simulink model "TSR_Scenario_006_cs"  (Simulink 7.6)
settings: Solver=ode5  SolverMode=SingleTasking  StartTime=0.0  StopTime=inf  FixedStep=1/100  RelTol=1e-3
model workspace (MAT data in the model file):
  mbox_table : struct (value not decoded)
  model_closed = 0
  sim_status = 0
PreLoadFcn:
  | check_NUTS_defined;
  | 
  | assignin('base',['model_closed_' bdroot],false);
  | 
  | addpath('../includes_TSR/includes_TSR');
  | 
  | switch version('-release')
  | case {'2010a', '2010b', '2011a'}
  | addpath('../includes_TSR/ML2010b');
  | otherwise
  | addpath('../includes_TSR/ML2011b');
  | end
InitFcn:
  | PreScanExperimentInitFcn(bdroot)
StopFcn:
  | PreScanExperimentStopFcn(bdroot)
undefined symbols (not defined in the file): DiscIntNeverNeededParam, InitImageOutputDir, x_ini_VRML, y_ini_VRML, z_ini_VRML
libraries: simulink x36, PreScanSimulinkLibrary x25, simulink_extras x18, PreScanUsefulBlocks x7, simulink_need_slupdate x1
(part 1 of 10)
CloseFcn:
  | evalin('base',['clear model_closed_' bdroot]);
settings Model: Creator=PRESCAN  LastModifiedBy=buildbot
settings OptimizationCC: InitFltsAndDblsToZero=on
settings DebuggingCC: SaveWithParameterizedLinksMsg=none  SignalResolutionControl=TryResolveAllWithWarning  SolverPrmCheckMsg=none  MultiTaskDSMMsg=warning  MultiTaskCondExecSysMsg=none
settings SFSimCC: SimParseCustomCode=off
settings RTWCC: IncludeERTFirstTime=on
settings GRTTargetCC: TargetFcnLib=ansi_tfl_tmw.mat

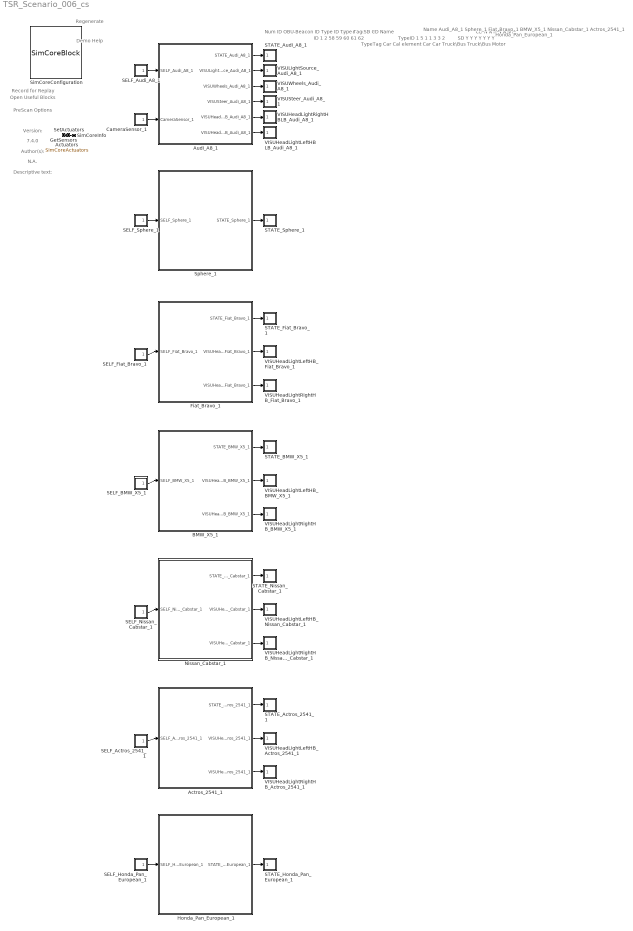
== system TSR_Scenario_006_cs ==
  note: Demo Help
  note: Regenerate
  note: Record for Replay
  note: Open Useful Blocks
  note: PreScan Options
  note: Version:
  note: 7.4.0
  note: Author(s):
  note: N.A.
  note: Descriptive text:
  note: ID
      |
      | 1
      | 2
      | 58
      | 59
      | 60
      | 61
      | 62
  note: OBU-Beacon ID
  note: TypeID
      |
      | 1
      | 5
      | 1
      | 1
      | 3
      | 3
      | 2
  note: TypeTag
      |
      | Car
      | Cal element
      | Car
      | Car
      | Truck\Bus
      | Truck\Bus
      | Motor
  note: SD
      |
      | Y
      | Y
      | Y
      | Y
      | Y
      | Y
      | Y
  note: CD
      |
      | N
      | N
      | N
      | N
      | N
      | N
      | N
  note: Name
      |
      | Audi_A8_1
      | Sphere_1
      | Fiat_Bravo_1
      | BMW_X5_1
      | Nissan_Cabstar_1
      | Actros_2541_1
      | Honda_Pan_European_1
  note: Num ID OBU-Beacon ID Type ID Type Tag SD CD Name
  Actros_2541_1 : Subsystem  Tag=WorldObjectSubSystem  InitFcn=UniqueId = '3230';
      mask Display: image(imread('Actros_2541.png'));color('white');text(0,0,' ID=61\n')
  Actuators : DataStoreMemory  Tag=Actuators  DataStoreName=SimCoreActuators  InitialValue=zeros(571,1)
      settings: DeleteFcn=PreScanBlockDeleteFcn;
  Audi_A8_1 : Subsystem  Tag=WorldObjectSubSystem  InitFcn=UniqueId = '253';
      mask Display: image(imread('Audi_A8.jpg'));color('white');text(0,0,' ID=1\n')
  BMW_X5_1 : Subsystem  Tag=WorldObjectSubSystem  InitFcn=UniqueId = '3222';
      mask Display: image(imread('BMW_X5.jpg'));color('white');text(0,0,' ID=59\n')
  CameraSensor_1 : Subsystem  Tag=CameraSensor  Priority=3
      settings: DeleteFcn=PreScanBlockDeleteFcn;
      mask Type: PreScan Source Block: Camera Sensor
      mask Description: The Camera Sensor provides a color or monochrome image.
      mask Help: eval('openHelp(457)')
      mask Display: image(imread('CameraSensor.png'))
  Fiat_Bravo_1 : Subsystem  Tag=WorldObjectSubSystem  InitFcn=UniqueId = '3219';
      mask Display: image(imread('Fiat_Bravo.jpg'));color('white');text(0,0,' ID=58\n')
  GetSensors : Subsystem  Tag=GetSensors  Priority=2  mask(PreScan Simulation Core Block){NrOfSensors=56, TimeStep=1/100}
      mask prompts: NrOfSensors "Number of sensor values"; TimeStep "Timestep [s]"
      mask help:
      | Please do not remove this block from the PreScan compilation sheet,
      | as it contains essential configuration parameters for a PreScan simulation.
      settings: DeleteFcn=PreScanBlockDeleteFcn;
  Honda_Pan_European_1 : Subsystem  Tag=WorldObjectSubSystem  InitFcn=UniqueId = '3233';
      mask Display: image(imread('Honda_Pan_European.jpg'));color('white');text(0,0,' ID=62\n')
  Nissan_Cabstar_1 : Subsystem  Tag=WorldObjectSubSystem  InitFcn=UniqueId = '3227';
      mask Display: image(imread('Nissan_Cabstar.jpg'));color('white');text(0,0,' ID=60\n')
  SELF_Actros_2541_1 : Subsystem  Tag=SELF  Priority=3  mask(PreScan Source Block: SELF){PortName=SELF_Actros_2541_1, PortIndex=40, PortWidth=8, TimeStep=1/100}
      mask prompts: PortName "Auto-Assigned: Port Name [-]"; PortIndex "Auto-Assigned: Port Index [-]"; PortWidth "Auto-Assigned: Port Dimensions"; TimeStep "Auto-Assigned: Upload Period [s]"
      mask help:
      | The SELF port shows (state) information of the actor itself. The outputs are position in the experiment's axis system and the GPS coordinates, and the object's absolute velocity and compass heading.
      |
      | For more information, please click Help.
      settings: DeleteFcn=PreScanBlockDeleteFcn;
      mask Help: eval('openHelp(462)')
      mask Display: image(imread('GPS.png'))
  SELF_Audi_A8_1 : Subsystem  Tag=SELF  Priority=3  mask(PreScan Source Block: SELF){PortName=SELF_Audi_A8_1, PortIndex=0, PortWidth=8, TimeStep=1/100}
      mask prompts: PortName "Auto-Assigned: Port Name [-]"; PortIndex "Auto-Assigned: Port Index [-]"; PortWidth "Auto-Assigned: Port Dimensions"; TimeStep "Auto-Assigned: Upload Period [s]"
      mask help:
      | The SELF port shows (state) information of the actor itself. The outputs are position in the experiment's axis system and the GPS coordinates, and the object's absolute velocity and compass heading.
      |
      | For more information, please click Help.
      settings: DeleteFcn=PreScanBlockDeleteFcn;
      mask Help: eval('openHelp(462)')
      mask Display: image(imread('GPS.png'))
  SELF_BMW_X5_1 : Subsystem  Tag=SELF  Priority=3  mask(PreScan Source Block: SELF){PortName=SELF_BMW_X5_1, PortIndex=24, PortWidth=8, TimeStep=1/100}
      mask prompts: PortName "Auto-Assigned: Port Name [-]"; PortIndex "Auto-Assigned: Port Index [-]"; PortWidth "Auto-Assigned: Port Dimensions"; TimeStep "Auto-Assigned: Upload Period [s]"
      mask help:
      | The SELF port shows (state) information of the actor itself. The outputs are position in the experiment's axis system and the GPS coordinates, and the object's absolute velocity and compass heading.
      |
      | For more information, please click Help.
      settings: DeleteFcn=PreScanBlockDeleteFcn;
      mask Help: eval('openHelp(462)')
      mask Display: image(imread('GPS.png'))
  SELF_Fiat_Bravo_1 : Subsystem  Tag=SELF  Priority=3  mask(PreScan Source Block: SELF){PortName=SELF_Fiat_Bravo_1, PortIndex=16, PortWidth=8, TimeStep=1/100}
      mask prompts: PortName "Auto-Assigned: Port Name [-]"; PortIndex "Auto-Assigned: Port Index [-]"; PortWidth "Auto-Assigned: Port Dimensions"; TimeStep "Auto-Assigned: Upload Period [s]"
      mask help:
      | The SELF port shows (state) information of the actor itself. The outputs are position in the experiment's axis system and the GPS coordinates, and the object's absolute velocity and compass heading.
      |
      | For more information, please click Help.
      settings: DeleteFcn=PreScanBlockDeleteFcn;
      mask Help: eval('openHelp(462)')
      mask Display: image(imread('GPS.png'))
  SELF_Honda_Pan_European_1 : Subsystem  Tag=SELF  Priority=3  mask(PreScan Source Block: SELF){PortName=SELF_Honda_Pan_European_1, PortIndex=48, PortWidth=8, TimeStep=1/100}
      mask prompts: PortName "Auto-Assigned: Port Name [-]"; PortIndex "Auto-Assigned: Port Index [-]"; PortWidth "Auto-Assigned: Port Dimensions"; TimeStep "Auto-Assigned: Upload Period [s]"
      mask help:
      | The SELF port shows (state) information of the actor itself. The outputs are position in the experiment's axis system and the GPS coordinates, and the object's absolute velocity and compass heading.
      |
      | For more information, please click Help.
      settings: DeleteFcn=PreScanBlockDeleteFcn;
      mask Help: eval('openHelp(462)')
      mask Display: image(imread('GPS.png'))
  SELF_Nissan_Cabstar_1 : Subsystem  Tag=SELF  Priority=3  mask(PreScan Source Block: SELF){PortName=SELF_Nissan_Cabstar_1, PortIndex=32, PortWidth=8, TimeStep=1/100}
      mask prompts: PortName "Auto-Assigned: Port Name [-]"; PortIndex "Auto-Assigned: Port Index [-]"; PortWidth "Auto-Assigned: Port Dimensions"; TimeStep "Auto-Assigned: Upload Period [s]"
      mask help:
      | The SELF port shows (state) information of the actor itself. The outputs are position in the experiment's axis system and the GPS coordinates, and the object's absolute velocity and compass heading.
      |
      | For more information, please click Help.
      settings: DeleteFcn=PreScanBlockDeleteFcn;
      mask Help: eval('openHelp(462)')
      mask Display: image(imread('GPS.png'))
  SELF_Sphere_1 : Subsystem  Tag=SELF  Priority=3  mask(PreScan Source Block: SELF){PortName=SELF_Sphere_1, PortIndex=8, PortWidth=8, TimeStep=1/100}
      mask prompts: PortName "Auto-Assigned: Port Name [-]"; PortIndex "Auto-Assigned: Port Index [-]"; PortWidth "Auto-Assigned: Port Dimensions"; TimeStep "Auto-Assigned: Upload Period [s]"
      mask help:
      | The SELF port shows (state) information of the actor itself. The outputs are position in the experiment's axis system and the GPS coordinates, and the object's absolute velocity and compass heading.
      |
      | For more information, please click Help.
      settings: DeleteFcn=PreScanBlockDeleteFcn;
      mask Help: eval('openHelp(462)')
      mask Display: image(imread('GPS.png'))
  STATE_Actros_2541_1 : Subsystem  Tag=State  Priority=0  mask(PreScan Sink Block: State){x0=-317.51490220295977, y0=442.15687795747425, z0=0.6, Roll0=0, Pitch0=0, Yaw0=329.99999999999994, TimeStep=1/100}
      mask prompts: x0 "Ini x-position VEHICLE wrt GLOBAL axis system [m]"; y0 "Ini y-position VEHICLE wrt GLOBAL axis system [m]"; z0 "Ini z-position VEHICLE wrt GLOBAL axis system [m]"; Roll0 "Ini roll-angle BODY wrt VEHICLE axis system [deg]"; Pitch0 "Ini pitch-angle BODY wrt VEHICLE axis system [deg]"; Yaw0 "Ini yaw-angle VEHICLE wrt GLOBAL axis system [deg]"; TimeStep "Time Step [s]"
      mask help:
      | The Actor State contains a vector signal of size (9x1), containing the following signals:
      |
      | -  Position                  (x,y,z)                                     [m]
      | -  Velocity                  (vx,vy,vz)                               [m/s]
      | -  Angles                    (Roll, Pitch, Yaw)                   [rad]
      |
      | The Actor state is defined in the global axis system.
      | The state is superponed on the Initial position defined in the GUI.
      |
      | For more information, please click Help.
      settings: DeleteFcn=PreScanBlockDeleteFcn;
      mask Help: eval('openHelp(222)')
      mask Display: image(imread('State.png'))
  STATE_Audi_A8_1 : Subsystem  Tag=State  Priority=0  mask(PreScan Sink Block: State){x0=-413.08909402600443, y0=672.31264940005644, z0=0.55, Roll0=0, Pitch0=0, Yaw0=19.15644857361562, TimeStep=1/100}
      mask prompts: x0 "Ini x-position VEHICLE wrt GLOBAL axis system [m]"; y0 "Ini y-position VEHICLE wrt GLOBAL axis system [m]"; z0 "Ini z-position VEHICLE wrt GLOBAL axis system [m]"; Roll0 "Ini roll-angle BODY wrt VEHICLE axis system [deg]"; Pitch0 "Ini pitch-angle BODY wrt VEHICLE axis system [deg]"; Yaw0 "Ini yaw-angle VEHICLE wrt GLOBAL axis system [deg]"; TimeStep "Time Step [s]"
      mask help:
      | The Actor State contains a vector signal of size (9x1), containing the following signals:
      |
      | -  Position                  (x,y,z)                                     [m]
      | -  Velocity                  (vx,vy,vz)                               [m/s]
      | -  Angles                    (Roll, Pitch, Yaw)                   [rad]
      |
      | The Actor state is defined in the global axis system.
      | The state is superponed on the Initial position defined in the GUI.
      |
      | For more information, please click Help.
      settings: DeleteFcn=PreScanBlockDeleteFcn;
      mask Help: eval('openHelp(222)')
      mask Display: image(imread('State.png'))
  STATE_BMW_X5_1 : Subsystem  Tag=State  Priority=0  mask(PreScan Sink Block: State){x0=-278.56622618717029, y0=100.14255486855011, z0=0.69, Roll0=0, Pitch0=0, Yaw0=248.31002382560104, TimeStep=1/100}
      mask prompts: x0 "Ini x-position VEHICLE wrt GLOBAL axis system [m]"; y0 "Ini y-position VEHICLE wrt GLOBAL axis system [m]"; z0 "Ini z-position VEHICLE wrt GLOBAL axis system [m]"; Roll0 "Ini roll-angle BODY wrt VEHICLE axis system [deg]"; Pitch0 "Ini pitch-angle BODY wrt VEHICLE axis system [deg]"; Yaw0 "Ini yaw-angle VEHICLE wrt GLOBAL axis system [deg]"; TimeStep "Time Step [s]"
      mask help:
      | The Actor State contains a vector signal of size (9x1), containing the following signals:
      |
      | -  Position                  (x,y,z)                                     [m]
      | -  Velocity                  (vx,vy,vz)                               [m/s]
      | -  Angles                    (Roll, Pitch, Yaw)                   [rad]
      |
      | The Actor state is defined in the global axis system.
      | The state is superponed on the Initial position defined in the GUI.
      |
      | For more information, please click Help.
      settings: DeleteFcn=PreScanBlockDeleteFcn;
      mask Help: eval('openHelp(222)')
      mask Display: image(imread('State.png'))
  STATE_Fiat_Bravo_1 : Subsystem  Tag=State  Priority=0  mask(PreScan Sink Block: State){x0=-278.56622618717029, y0=100.14255486855011, z0=0.55, Roll0=0, Pitch0=0, Yaw0=248.31002382560104, TimeStep=1/100}
      mask prompts: x0 "Ini x-position VEHICLE wrt GLOBAL axis system [m]"; y0 "Ini y-position VEHICLE wrt GLOBAL axis system [m]"; z0 "Ini z-position VEHICLE wrt GLOBAL axis system [m]"; Roll0 "Ini roll-angle BODY wrt VEHICLE axis system [deg]"; Pitch0 "Ini pitch-angle BODY wrt VEHICLE axis system [deg]"; Yaw0 "Ini yaw-angle VEHICLE wrt GLOBAL axis system [deg]"; TimeStep "Time Step [s]"
      mask help:
      | The Actor State contains a vector signal of size (9x1), containing the following signals:
      |
      | -  Position                  (x,y,z)                                     [m]
      | -  Velocity                  (vx,vy,vz)                               [m/s]
      | -  Angles                    (Roll, Pitch, Yaw)                   [rad]
      |
      | The Actor state is defined in the global axis system.
      | The state is superponed on the Initial position defined in the GUI.
      |
      | For more information, please click Help.
      settings: DeleteFcn=PreScanBlockDeleteFcn;
      mask Help: eval('openHelp(222)')
      mask Display: image(imread('State.png'))
  STATE_Honda_Pan_European_1 : Subsystem  Tag=State  Priority=0  mask(PreScan Sink Block: State){x0=-295.55667114257812, y0=275.828369140625, z0=0.594, Roll0=0, Pitch0=0, Yaw0=330, TimeStep=1/100}
      mask prompts: x0 "Ini x-position VEHICLE wrt GLOBAL axis system [m]"; y0 "Ini y-position VEHICLE wrt GLOBAL axis system [m]"; z0 "Ini z-position VEHICLE wrt GLOBAL axis system [m]"; Roll0 "Ini roll-angle BODY wrt VEHICLE axis system [deg]"; Pitch0 "Ini pitch-angle BODY wrt VEHICLE axis system [deg]"; Yaw0 "Ini yaw-angle VEHICLE wrt GLOBAL axis system [deg]"; TimeStep "Time Step [s]"
      mask help:
      | The Actor State contains a vector signal of size (9x1), containing the following signals:
      |
      | -  Position                  (x,y,z)                                     [m]
      | -  Velocity                  (vx,vy,vz)                               [m/s]
      | -  Angles                    (Roll, Pitch, Yaw)                   [rad]
      |
      | The Actor state is defined in the global axis system.
      | The state is superponed on the Initial position defined in the GUI.
      |
      | For more information, please click Help.
      settings: DeleteFcn=PreScanBlockDeleteFcn;
      mask Help: eval('openHelp(222)')
      mask Display: image(imread('State.png'))
  STATE_Nissan_Cabstar_1 : Subsystem  Tag=State  Priority=0  mask(PreScan Sink Block: State){x0=-125.23931337038341, y0=335.18796687071978, z0=0.88, Roll0=0, Pitch0=0, Yaw0=150, TimeStep=1/100}
      mask prompts: x0 "Ini x-position VEHICLE wrt GLOBAL axis system [m]"; y0 "Ini y-position VEHICLE wrt GLOBAL axis system [m]"; z0 "Ini z-position VEHICLE wrt GLOBAL axis system [m]"; Roll0 "Ini roll-angle BODY wrt VEHICLE axis system [deg]"; Pitch0 "Ini pitch-angle BODY wrt VEHICLE axis system [deg]"; Yaw0 "Ini yaw-angle VEHICLE wrt GLOBAL axis system [deg]"; TimeStep "Time Step [s]"
      mask help:
      | The Actor State contains a vector signal of size (9x1), containing the following signals:
      |
      | -  Position                  (x,y,z)                                     [m]
      | -  Velocity                  (vx,vy,vz)                               [m/s]
      | -  Angles                    (Roll, Pitch, Yaw)                   [rad]
      |
      | The Actor state is defined in the global axis system.
      | The state is superponed on the Initial position defined in the GUI.
      |
      | For more information, please click Help.
      settings: DeleteFcn=PreScanBlockDeleteFcn;
      mask Help: eval('openHelp(222)')
      mask Display: image(imread('State.png'))
  STATE_Sphere_1 : Subsystem  Tag=State  Priority=0  mask(PreScan Sink Block: State){x0=-413.089094026004, y0=672.312649400056, z0=0.55, Roll0=0, Pitch0=0, Yaw0=19.1564485736156, TimeStep=1/100}
      mask prompts: x0 "Ini x-position VEHICLE wrt GLOBAL axis system [m]"; y0 "Ini y-position VEHICLE wrt GLOBAL axis system [m]"; z0 "Ini z-position VEHICLE wrt GLOBAL axis system [m]"; Roll0 "Ini roll-angle BODY wrt VEHICLE axis system [deg]"; Pitch0 "Ini pitch-angle BODY wrt VEHICLE axis system [deg]"; Yaw0 "Ini yaw-angle VEHICLE wrt GLOBAL axis system [deg]"; TimeStep "Time Step [s]"
      mask help:
      | The Actor State contains a vector signal of size (9x1), containing the following signals:
      |
      | -  Position                  (x,y,z)                                     [m]
      | -  Velocity                  (vx,vy,vz)                               [m/s]
      | -  Angles                    (Roll, Pitch, Yaw)                   [rad]
      |
      | The Actor state is defined in the global axis system.
      | The state is superponed on the Initial position defined in the GUI.
      |
      | For more information, please click Help.
      settings: DeleteFcn=PreScanBlockDeleteFcn;
      mask Help: eval('openHelp(222)')
      mask Display: image(imread('State.png'))
  SetActuators : Subsystem  Tag=SetActuators  Priority=1  mask(PreScan Simulation Core Block){TimeStep=1/100, NrOfActuators=571}
      mask prompts: TimeStep "Timestep [s]"; NrOfActuators "Number of actuator values"
      mask help:
      | Please do not remove this block from the PreScan compilation sheet,
      | as it contains essential configuration parameters for a PreScan simulation.
      settings: DeleteFcn=PreScanBlockDeleteFcn;
  SimCoreConfiguration : M-S-Function  Tag=SimCoreConfiguration  Description=313268978F12D5AD1759FB37E42A829EE63F37BD296FA7458A7FCDBDC14E6B1E  FunctionName=SimCoreBlock  Parameters=ExperimentXML PortsXML SimulationCore HostName CheckStart EnableLog RfR EnableGPUAccel ShowComputationTime  mask(PreScan Simulation Core Configurator){SimulationCore=NUTS, HostName=0, CheckStart=0, prescanversion='7.4.0', EnableLog=off, RfR=0, EnableGPUAccel=off, ShowComputationTime=off}
      mask prompts: SimulationCore "Simulation Core"; HostName "Simulation Host"; CheckStart "Show START Dialog"; prescanversion "PreScan Version"; EnableLog "Create TA Log"; RfR "Record for Replay"; EnableGPUAccel "Enable GPU Acceleration"; ShowComputationTime "Show ComputationTime Scope"
      mask help:
      | Please do not remove this block from the PreScan compilation sheet,
      | as it contains essential configuration parameter for a PreScan simulation.
      mask init:
      | model = bdroot;
      | ExperimentXML = [model(1:end-3) '.pex'];
      | PortsXML = [model '_ports.pcd'];
      settings: DeleteFcn=PreScanBlockDeleteFcn;  ModelCloseFcn=assignin('base',['model_closed_' bdroot],true);
      mask Help: eval('openHelp(812)')
      mask Display: image(imread('prescanlogo.ico'))
  SimCoreInfo : Subsystem  Tag=SimCoreInfo
  Sphere_1 : Subsystem  Tag=WorldObjectSubSystem  InitFcn=UniqueId = '277';
      mask Display: image(imread('Sphere.jpg'));color('white');text(0,0,' ID=2\n')
  VISUHeadLightLeftHBLB_Audi_A8_1 : Subsystem  Tag=VisuLights  Priority=0
      settings: DeleteFcn=PreScanBlockDeleteFcn;
      mask Type: PreScan Sink Block: VisuLights
      mask Description:
      | The VisuLights block provides a way to animate the active lights of a vehicle with possibilities to adapt the:
      | - Intensity [-]
      | - Position (x,y,z) [m]
      | - Orientation (Roll, Pitch, Yaw) [deg]
      | - Color (RGB) [-]
      | - TextureResourceID [-]
      | 
      | For more information, please click Help.
      mask Help: eval('openHelp(231)')
      mask Display: image(imread('HeadLight.png'))
  VISUHeadLightLeftHB_Actros_2541_1 : Subsystem  Tag=VisuLights  Priority=0
      settings: DeleteFcn=PreScanBlockDeleteFcn;
      mask Type: PreScan Sink Block: VisuLights
      mask Description:
      | The VisuLights block provides a way to animate the active lights of a vehicle with possibilities to adapt the:
      | - Intensity [-]
      | - Position (x,y,z) [m]
      | - Orientation (Roll, Pitch, Yaw) [deg]
      | - Color (RGB) [-]
      | - TextureResourceID [-]
      | 
      | For more information, please click Help.
      mask Help: eval('openHelp(231)')
      mask Display: image(imread('HeadLight.png'))
  VISUHeadLightLeftHB_BMW_X5_1 : Subsystem  Tag=VisuLights  Priority=0
      settings: DeleteFcn=PreScanBlockDeleteFcn;
      mask Type: PreScan Sink Block: VisuLights
      mask Description:
      | The VisuLights block provides a way to animate the active lights of a vehicle with possibilities to adapt the:
      | - Intensity [-]
      | - Position (x,y,z) [m]
      | - Orientation (Roll, Pitch, Yaw) [deg]
      | - Color (RGB) [-]
      | - TextureResourceID [-]
      | 
      | For more information, please click Help.
      mask Help: eval('openHelp(231)')
      mask Display: image(imread('HeadLight.png'))
  VISUHeadLightLeftHB_Fiat_Bravo_1 : Subsystem  Tag=VisuLights  Priority=0
      settings: DeleteFcn=PreScanBlockDeleteFcn;
      mask Type: PreScan Sink Block: VisuLights
      mask Description:
      | The VisuLights block provides a way to animate the active lights of a vehicle with possibilities to adapt the:
      | - Intensity [-]
      | - Position (x,y,z) [m]
      | - Orientation (Roll, Pitch, Yaw) [deg]
      | - Color (RGB) [-]
      | - TextureResourceID [-]
      | 
      | For more information, please click Help.
      mask Help: eval('openHelp(231)')
      mask Display: image(imread('HeadLight.png'))
  VISUHeadLightLeftHB_Nissan_Cabstar_1 : Subsystem  Tag=VisuLights  Priority=0
      settings: DeleteFcn=PreScanBlockDeleteFcn;
      mask Type: PreScan Sink Block: VisuLights
      mask Description:
      | The VisuLights block provides a way to animate the active lights of a vehicle with possibilities to adapt the:
      | - Intensity [-]
      | - Position (x,y,z) [m]
      | - Orientation (Roll, Pitch, Yaw) [deg]
      | - Color (RGB) [-]
      | - TextureResourceID [-]
      | 
      | For more information, please click Help.
      mask Help: eval('openHelp(231)')
      mask Display: image(imread('HeadLight.png'))
  VISUHeadLightRightHBLB_Audi_A8_1 : Subsystem  Tag=VisuLights  Priority=0
      settings: DeleteFcn=PreScanBlockDeleteFcn;
      mask Type: PreScan Sink Block: VisuLights
      mask Description:
      | The VisuLights block provides a way to animate the active lights of a vehicle with possibilities to adapt the:
      | - Intensity [-]
      | - Position (x,y,z) [m]
      | - Orientation (Roll, Pitch, Yaw) [deg]
      | - Color (RGB) [-]
      | - TextureResourceID [-]
      | 
      | For more information, please click Help.
      mask Help: eval('openHelp(231)')
      mask Display: image(imread('HeadLight.png'))
  VISUHeadLightRightHB_Actros_2541_1 : Subsystem  Tag=VisuLights  Priority=0
      settings: DeleteFcn=PreScanBlockDeleteFcn;
      mask Type: PreScan Sink Block: VisuLights
      mask Description:
      | The VisuLights block provides a way to animate the active lights of a vehicle with possibilities to adapt the:
      | - Intensity [-]
      | - Position (x,y,z) [m]
      | - Orientation (Roll, Pitch, Yaw) [deg]
      | - Color (RGB) [-]
      | - TextureResourceID [-]
      | 
      | For more information, please click Help.
      mask Help: eval('openHelp(231)')
      mask Display: image(imread('HeadLight.png'))
  VISUHeadLightRightHB_BMW_X5_1 : Subsystem  Tag=VisuLights  Priority=0
      settings: DeleteFcn=PreScanBlockDeleteFcn;
      mask Type: PreScan Sink Block: VisuLights
      mask Description:
      | The VisuLights block provides a way to animate the active lights of a vehicle with possibilities to adapt the:
      | - Intensity [-]
      | - Position (x,y,z) [m]
      | - Orientation (Roll, Pitch, Yaw) [deg]
      | - Color (RGB) [-]
      | - TextureResourceID [-]
      | 
      | For more information, please click Help.
      mask Help: eval('openHelp(231)')
      mask Display: image(imread('HeadLight.png'))
  VISUHeadLightRightHB_Fiat_Bravo_1 : Subsystem  Tag=VisuLights  Priority=0
      settings: DeleteFcn=PreScanBlockDeleteFcn;
      mask Type: PreScan Sink Block: VisuLights
      mask Description:
      | The VisuLights block provides a way to animate the active lights of a vehicle with possibilities to adapt the:
      | - Intensity [-]
      | - Position (x,y,z) [m]
      | - Orientation (Roll, Pitch, Yaw) [deg]
      | - Color (RGB) [-]
      | - TextureResourceID [-]
      | 
      | For more information, please click Help.
      mask Help: eval('openHelp(231)')
      mask Display: image(imread('HeadLight.png'))
  VISUHeadLightRightHB_Nissan_Cabstar_1 : Subsystem  Tag=VisuLights  Priority=0
      settings: DeleteFcn=PreScanBlockDeleteFcn;
      mask Type: PreScan Sink Block: VisuLights
      mask Description:
      | The VisuLights block provides a way to animate the active lights of a vehicle with possibilities to adapt the:
      | - Intensity [-]
      | - Position (x,y,z) [m]
      | - Orientation (Roll, Pitch, Yaw) [deg]
      | - Color (RGB) [-]
      | - TextureResourceID [-]
      | 
      | For more information, please click Help.
      mask Help: eval('openHelp(231)')
      mask Display: image(imread('HeadLight.png'))
  VISULightSource_Audi_A8_1 : Subsystem  Tag=VisuLightSource  Priority=0
      settings: DeleteFcn=PreScanBlockDeleteFcn;
      mask Type: PreScan Sink Block: VisuLightSource
      mask Description:
      | The VisuLightSource block provides a way to animate Light Sources of the indicator, braking, fog and main lights of a vehicle.
      | 
      | For more information, please click Help.
      mask Help: eval('openHelp(223)')
      mask Display: image(imread('RearLight.png'))
  VISUSteer_Audi_A8_1 : Subsystem  Tag=VisuSteer  Priority=0
      settings: DeleteFcn=PreScanBlockDeleteFcn;
      mask Type: PreScan Sink Block: VisuSteer
      mask Description:
      | The VisuSteer block provides a way to adapt the orientation of the steering column and steering wheel of a vehicle.
      | 
      | For more information, please click Help.
      mask Help: eval('openHelp(223)')
      mask Display: image(imread('steeringwheel.png'))
  VISUWheels_Audi_A8_1 : Subsystem  Tag=VisuWheels  Priority=0
      settings: DeleteFcn=PreScanBlockDeleteFcn;
      mask Type: PreScan Sink Block: VisuWheels
      mask Description:
      | The VisuWheels block provides a way to animate the wheels of a vehicle, with steering, rotation (because of velocity) and z-displacement.
      | 
      | For more information, please click Help.
      mask Help: eval('openHelp(223)')
      mask Display: image(imread('wheel.png'))
  wires:
  Audi_A8_1/1(STATE_Audi_A8_1) -> STATE_Audi_A8_1/1(State)
  SELF_Audi_A8_1/1(U) -> Audi_A8_1/1(SELF_Audi_A8_1)
  CameraSensor_1/1(U1) -> Audi_A8_1/2(CameraSensor_1)
  Audi_A8_1/2(VISULightSource_Audi_A8_1) -> VISULightSource_Audi_A8_1/1(Lights)
  Audi_A8_1/3(VISUWheels_Audi_A8_1) -> VISUWheels_Audi_A8_1/1(Wheels)
  Audi_A8_1/4(VISUSteer_Audi_A8_1) -> VISUSteer_Audi_A8_1/1(Steer)
  Audi_A8_1/5(VISUHeadLightRightHBLB_Audi_A8_1) -> VISUHeadLightRightHBLB_Audi_A8_1/1(Lights)
  Audi_A8_1/6(VISUHeadLightLeftHBLB_Audi_A8_1) -> VISUHeadLightLeftHBLB_Audi_A8_1/1(Lights)
  Sphere_1/1(STATE_Sphere_1) -> STATE_Sphere_1/1(State)
  SELF_Sphere_1/1(U) -> Sphere_1/1(SELF_Sphere_1)
  Fiat_Bravo_1/1(STATE_Fiat_Bravo_1) -> STATE_Fiat_Bravo_1/1(State)
  SELF_Fiat_Bravo_1/1(U) -> Fiat_Bravo_1/1(SELF_Fiat_Bravo_1)
  Fiat_Bravo_1/2(VISUHeadLightLeftHB_Fiat_Bravo_1) -> VISUHeadLightLeftHB_Fiat_Bravo_1/1(Lights)
  Fiat_Bravo_1/3(VISUHeadLightRightHB_Fiat_Bravo_1) -> VISUHeadLightRightHB_Fiat_Bravo_1/1(Lights)
  BMW_X5_1/1(STATE_BMW_X5_1) -> STATE_BMW_X5_1/1(State)
  SELF_BMW_X5_1/1(U) -> BMW_X5_1/1(SELF_BMW_X5_1)
  BMW_X5_1/2(VISUHeadLightLeftHB_BMW_X5_1) -> VISUHeadLightLeftHB_BMW_X5_1/1(Lights)
  BMW_X5_1/3(VISUHeadLightRightHB_BMW_X5_1) -> VISUHeadLightRightHB_BMW_X5_1/1(Lights)
  Nissan_Cabstar_1/1(STATE_Nissan_Cabstar_1) -> STATE_Nissan_Cabstar_1/1(State)
  SELF_Nissan_Cabstar_1/1(U) -> Nissan_Cabstar_1/1(SELF_Nissan_Cabstar_1)
  Nissan_Cabstar_1/2(VISUHeadLightLeftHB_Nissan_Cabstar_1) -> VISUHeadLightLeftHB_Nissan_Cabstar_1/1(Lights)
  Nissan_Cabstar_1/3(VISUHeadLightRightHB_Nissan_Cabstar_1) -> VISUHeadLightRightHB_Nissan_Cabstar_1/1(Lights)
  Actros_2541_1/1(STATE_Actros_2541_1) -> STATE_Actros_2541_1/1(State)
  SELF_Actros_2541_1/1(U) -> Actros_2541_1/1(SELF_Actros_2541_1)
  Actros_2541_1/2(VISUHeadLightLeftHB_Actros_2541_1) -> VISUHeadLightLeftHB_Actros_2541_1/1(Lights)
  Actros_2541_1/3(VISUHeadLightRightHB_Actros_2541_1) -> VISUHeadLightRightHB_Actros_2541_1/1(Lights)
  Honda_Pan_European_1/1(STATE_Honda_Pan_European_1) -> STATE_Honda_Pan_European_1/1(State)
  SELF_Honda_Pan_European_1/1(U) -> Honda_Pan_European_1/1(SELF_Honda_Pan_European_1)
  SetActuators/1(dummy) -> GetSensors/1(dummy)

== system TSR_Scenario_006_cs/Actros_2541_1 ==
  note: Resources
      |
      | 1: LightMap\HeadLight LB and HB.png: HeadLight LB and HB
      | 2: LightMap\HeadLight HB.png: HeadLight HB
  note: Resources
  SELF_Actros_2541_1 : Inport  Tag=SELFInport
  HeadLightLeftHB_Col : Constant  Tag=VisuLightConst  Value=[255 249 224]
  HeadLightLeftHB_ID : Constant  Tag=VisuLightConst  Value=[0]
  HeadLightLeftHB_Ori : Constant  Tag=VisuLightConst  Value=[0 2 358]
  HeadLightLeftHB_Pos : Constant  Tag=VisuLightConst  Value=[5.93481 1.00553 0.797323]
  HeadLightLeftHB_mscd : Constant  Tag=VisuLightConst  Value=[98.20]
  HeadLightRightHB_Col : Constant  Tag=VisuLightConst  Value=[255 249 224]
  HeadLightRightHB_ID : Constant  Tag=VisuLightConst  Value=[0]
  HeadLightRightHB_Ori : Constant  Tag=VisuLightConst  Value=[0 0 358]
  HeadLightRightHB_Pos : Constant  Tag=VisuLightConst  Value=[5.93481 -1.0055 0.797323]
  HeadLightRightHB_mscd : Constant  Tag=VisuLightConst  Value=[98.20]
  SELF_Demux : Subsystem  Tag=DemuxSELF
      settings: DeleteFcn=PreScanBlockDeleteFcn;
      mask Type: PreScan Demux Block:
      mask Display:
      | port_label('output',1,'x [m]')
      | port_label('output',2,'y [m]')
      | port_label('output',3,'z [m]','texmode','on')
      | port_label('output',4,'Rotx [deg]','texmode','on')
      | port_label('output',5,'Roty [deg]','texmode','on')
      | port_label('output',6,'Rotz [deg]','texmode','on')
      | port_label('output',7,'GPS lat [deg]','texmode','on')
      | port_label('output',8,'GPS long [deg]','texmode','on')
      | port_label('output',9,'GPS alt [m]','texmode','on')
      | port_label('output',10,'Velocity [m/s]')
      | port_label('output',11,'Heading [deg]')
      | port_label('output',12,'Yaw rate [deg/s]')
  Terminator_{1..12} (12 alike) : Terminator
  Trajectories : Subsystem  Tag=Trajectories
      settings: DeleteFcn=PreScanBlockDeleteFcn;
      mask Type: PreScan Source Block: Trajectories
      mask Description:
      | The Trajectory block contains the trajectories defined in the PreScan Experiment Editor. The output of the trajectory block is the (vehicle) State.
      | 
      | For more information, please click Help.
      mask Help: eval('openHelp(312)')
      mask Display: image(imread('Trajectory.png'));
  VISUHeadLightLeftHB_Mux : Subsystem  Tag=MuxLights
      settings: DeleteFcn=PreScanBlockDeleteFcn;
      mask Type: PreScan Mux Block:
  VISUHeadLightRightHB_Mux : Subsystem  Tag=MuxLights
      settings: DeleteFcn=PreScanBlockDeleteFcn;
      mask Type: PreScan Mux Block:
  STATE_Actros_2541_1 : Outport  Tag=StateOutport
  VISUHeadLightLeftHB_Actros_2541_1 : Outport  Tag=VisuHeadLightLeftHBOutport  Port=2  SampleTime=1/100
  VISUHeadLightRightHB_Actros_2541_1 : Outport  Tag=VisuHeadLightRightHBOutport  Port=3  SampleTime=1/100
  wires:
  SELF_Actros_2541_1/1 -> SELF_Demux/1(SELF)
  VISUHeadLightLeftHB_Mux/1(Lights) -> VISUHeadLightLeftHB_Actros_2541_1/1
  HeadLightLeftHB_mscd/1 -> VISUHeadLightLeftHB_Mux/1(MSCD [Cd])
  HeadLightLeftHB_Pos/1 -> VISUHeadLightLeftHB_Mux/2(Position (xyz) [m])
  HeadLightLeftHB_Ori/1 -> VISUHeadLightLeftHB_Mux/3(Orientation (RPY) [deg])
  HeadLightLeftHB_Col/1 -> VISUHeadLightLeftHB_Mux/4(Color [-])
  HeadLightLeftHB_ID/1 -> VISUHeadLightLeftHB_Mux/5(TextureResourceID [-])
  VISUHeadLightRightHB_Mux/1(Lights) -> VISUHeadLightRightHB_Actros_2541_1/1
  HeadLightRightHB_mscd/1 -> VISUHeadLightRightHB_Mux/1(MSCD [Cd])
  HeadLightRightHB_Pos/1 -> VISUHeadLightRightHB_Mux/2(Position (xyz) [m])
  HeadLightRightHB_Ori/1 -> VISUHeadLightRightHB_Mux/3(Orientation (RPY) [deg])
  HeadLightRightHB_Col/1 -> VISUHeadLightRightHB_Mux/4(Color [-])
  HeadLightRightHB_ID/1 -> VISUHeadLightRightHB_Mux/5(TextureResourceID [-])
  Trajectories/1(State) -> STATE_Actros_2541_1/1
  SELF_Demux/1(x [m]) -> Terminator_1/1
  SELF_Demux/2(y [m]) -> Terminator_2/1
  SELF_Demux/3(z [m]) -> Terminator_3/1
  SELF_Demux/4(rotx [deg]) -> Terminator_4/1
  SELF_Demux/5(roty [deg]) -> Terminator_5/1
  SELF_Demux/6(rotz [deg]) -> Terminator_6/1
  SELF_Demux/7(GPS lat [deg]) -> Terminator_7/1
  SELF_Demux/8(GPS long [deg]) -> Terminator_8/1
  SELF_Demux/9(GPS alt [m]) -> Terminator_9/1
  SELF_Demux/10(velocity [m/s]) -> Terminator_10/1
  SELF_Demux/11(heading [deg]) -> Terminator_11/1
  SELF_Demux/12(yaw rate [deg/s]) -> Terminator_12/1

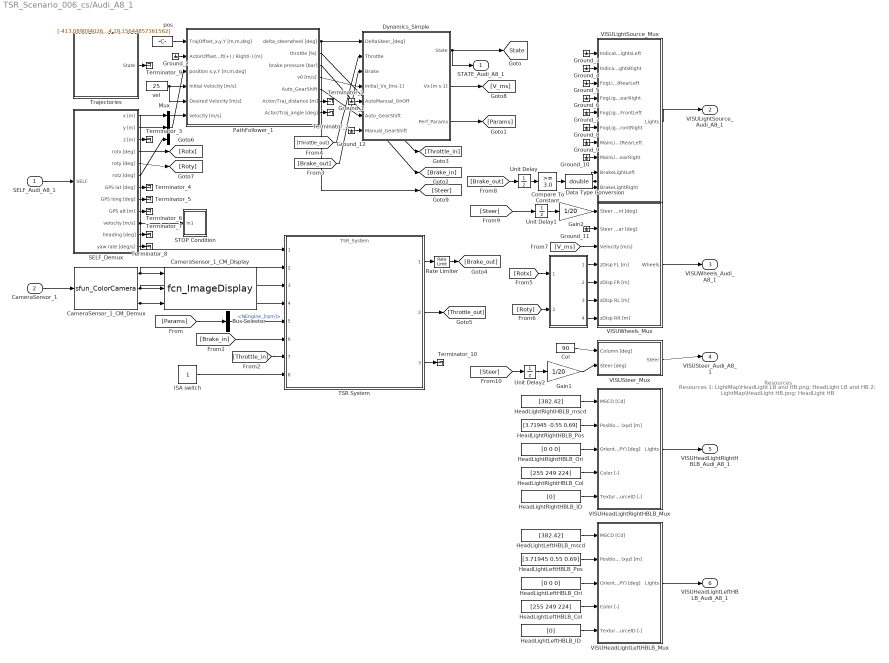
== system TSR_Scenario_006_cs/Audi_A8_1 ==
  note: Resources
      |
      | 1: LightMap\HeadLight LB and HB.png: HeadLight LB and HB
      | 2: LightMap\HeadLight HB.png: HeadLight HB
  note: Resources
  SELF_Audi_A8_1 : Inport  Tag=SELFInport
  CameraSensor_1 : Inport  Tag=CameraSensorInport  Port=2  SampleTime=1/50
  " " : Subsystem  mask{da=1.17, db=1.77, h=0.21, w=1.612}
      mask prompts: da "Distance to the front wheel from cars center of gravity [m]"; db "Distance to the back wheel from cars center of gravity [m]"; h "Center of gravity height [m]"; w "Width of the car [m]"
      mask init:
      | a  = sqrt( da*da + h*h );
      | b  = sqrt( db*db + h*h );
      | TW = sqrt( 0.25*w*w + h*h );
  Bus Selector : BusSelector  OutputSignals=NEngine_[rpm]
  CameraSensor_1_CM_Demux : S-Function  Tag=CameraSensor_Color_Demux  FunctionName=sfun_ColorCamera  Parameters=[VerticalResolution HorizontalResolution] FrameRate SensorName CameraType SharedMemTag SharedMemRightTag DataType  EnableBusSupport=off  mask{HorizontalResolution=800, VerticalResolution=600, FrameRate=50, SensorName=CameraSensor_1, CameraType=Mono, SharedMemTag=CameraSensor_1_monoBeam_viewer_RGB, SharedMemRightTag=CameraSensor_1_StereoRight_viewer_RGB, DataType=uint8}
      mask prompts: HorizontalResolution "User Specified: Horizontal Resolution [pixels]"; VerticalResolution "User Specified: Vertical Resolution [pixels]"; FrameRate "User Specified: Frame Rate [Hz]"; SensorName "User Specified: Camera Sensor Name"; CameraType "Camera Type"; SharedMemTag "Tag for shared memory for main img"; SharedMemRightTag "Tag for shared memory for right img"; DataType "Image Data Type"
      mask init:
      | if CameraType==1
      |     CameraTypeName='MONO';
      |     PortNumber=0;
      | else
      |     CameraTypeName='STEREO';
      |     PortNumber=3;
      | end
      settings: DeleteFcn=PreScanBlockDeleteFcn;
      mask StyleString: edit,edit,edit,edit,popup(Mono|Stereo),edit,edit,popup(uint8|single)
      mask Display:
      | fprintf('%s CAMERA:\n Color\n %s \n V: %d x %d \n %d fps',CameraTypeName,SensorName,VerticalResolution,HorizontalResolution,FrameRate)
      | port_label('output',1,'R')
      | port_label('output',2,'G')
      | port_label('output',3,'B')
      | port_label('output',PortNumber+1,'R')
      | port_label('output',PortNumber+2,'G')
      | port_label('output',PortNumber+3,'B')
  CameraSensor_1_CM_Display : M-S-Function  Tag=CameraSensor_Color_Display  InitFcn=InitImageOutputDir(gcb);  FunctionName=fcn_ImageDisplay  Parameters=SensorName EnableDisplay EnablePosition DisplayPosition FigureHandle SaveResults BitmapFormat TempOutputDir CameraType DataType  mask(PreScan Color Display Block){SensorName=CameraSensor_1, EnableDisplay=on, EnablePosition=off, DisplayPosition=[10 10 800 600], FigureHandle=100, SaveResults=off, Format=PNG, TempOutputDir=0, CameraType=Mono, DataType=uint8}
      mask prompts: SensorName "User Specified: Title of Display"; EnableDisplay "Active"; EnablePosition "Set Display window position"; DisplayPosition "Display window position [xpos ypos width height]"; FigureHandle "Unique Handle"; SaveResults "Save results"; TempOutputDir "OutputDir"; CameraType "Camera Type"; DataType "Image Data Type"
      mask help: This block displays the RGB output of a PreScan camera sensor.
      mask init:
      | if EnableDisplay
      |     EnableString='';
      |     EnableColor='gray';
      | else
      |     EnableString='INACTIVE';
      |     EnableColor='red';
      | end
      | switch Format
      |     case 1
      |         BitmapFormat = 'png';
      |     case 2
      |         BitmapFormat = 'bmp';
      |     case 3
      |         BitmapFormat = 'jpg';
      | end 
      | if CameraType==1
      |     CameraTypeName='MONO';
      |     PortNumber=0;
      | else
      |     CameraTypeName='STEREO';
      |     PortNumber=3;
      | end
      settings: CopyFcn=CopyFcnDisplay  DeleteFcn=PreScanBlockDeleteFcn;  ModelCloseFcn=fcn_ImageDisplay_ModelCloseFcn
      mask Help: eval('openHelp(457)')
      mask StyleString: edit,checkbox,checkbox,edit,edit,checkbox,popup(PNG|BMP|JPG),edit,popup(Mono|Stereo),popup(uint8|single)
      mask CallbackString:
      | ||MV=get_param(gcb,'MaskVisibilities');
      | if strcmp(get_param(gcb,'EnablePosition'),'on')
      |     MV{4}='on';
      | else
      |     MV{4}='off';
      | end
      | set_param(gcb,'MaskVisibilities',MV);|||||||
      mask Display:
      | color(EnableColor);
      | fprintf('%s\n DISPLAY:\n Color \n %s',EnableString,SensorName)
      | port_label('input',1,'R')
      | port_label('input',2,'G')
      | port_label('input',3,'B')
      | port_label('input',PortNumber+1,'R')
      | port_label('input',PortNumber+2,'G')
      | port_label('input',PortNumber+3,'B')
  Col : Constant  Value=90
  Compare To Constant : simulink/Logic and Bit Operations/Compare To Constant  SystemSampleTime=-1  relop=>=  const=3.0  LogicOutDataTypeMode=boolean
  Data Type Conversion : DataTypeConversion  OutDataTypeStr=double
  Dynamics_Simple : Subsystem  Tag=Simple_Vehicle_Dynamics  mask(PreScan Block: Simple Dynamics){Migrate=off, TimeStep=1/100, ComputationMode=Continuous_Time}
      mask prompts: Migrate "Migrate. During migration this block will be replaced by a newer one."; TimeStep "Auto assigned: Time Step [s]"; ComputationMode "Computation mode:"
      mask help:
      | The Simple Dynamics Model is selected in the GUI to simulate vehicle dynamics behavior.
      |
      | The Simple Dynamics Model is completely open to the user. The parameters of this model can be set in the Simple Dynamics dialog in the GUI.
      |
      | For more information, please click Help.
      mask init:
      | p = SimpleDyn_pars;
      settings: DeleteFcn=PreScanBlockDeleteFcn;
      mask Help: eval('openHelp(220)')
      mask Display:
      | image(imread('SimpleDyn.png'))
      | port_label('input', 1, '{\delta}_S_t_ _e_e_r [deg]','texmode','on')
      | port_label('input', 2, 'Throttle [%]')
      | port_label('input', 3, 'Brake Pres [bar]')
      | port_label('input', 4, 'V_0 [ms-1]','texmode','on')
      | port_label('input', 5, 'Auto=[0]/Manual=[1]')
      | port_label('input', 6, 'Auto_GearShift')
      | port_label('input', 7, 'Manual_GearShift')
      | port_label('output', 1, 'State')
      | port_label('output', 2, 'Vx [ms-1]')
      | port_label('output', 3, 'Perf Params')
  Gain1 : Gain  Gain=1/20
  Gain2 : Gain  Gain=1/20
  Ground_{1..12} (12 alike) : Ground
  HeadLightLeftHBLB_Col : Constant  Tag=VisuLightConst  Value=[255 249 224]
  HeadLightLeftHBLB_ID : Constant  Tag=VisuLightConst  Value=[0]
  HeadLightLeftHBLB_Ori : Constant  Tag=VisuLightConst  Value=[0 0 0]
  HeadLightLeftHBLB_Pos : Constant  Tag=VisuLightConst  Value=[3.71945 0.55 0.69]
  HeadLightLeftHBLB_mscd : Constant  Tag=VisuLightConst  Value=[382.42]
  HeadLightRightHBLB_Col : Constant  Tag=VisuLightConst  Value=[255 249 224]
  HeadLightRightHBLB_ID : Constant  Tag=VisuLightConst  Value=[0]
  HeadLightRightHBLB_Ori : Constant  Tag=VisuLightConst  Value=[0 0 0]
  HeadLightRightHBLB_Pos : Constant  Tag=VisuLightConst  Value=[3.71945 -0.55 0.69]
  HeadLightRightHBLB_mscd : Constant  Tag=VisuLightConst  Value=[382.42]
  ISA switch : Constant
  Mux : Mux  Inputs=3
  PathFollower_1 : Subsystem  Tag=pathFollower  mask(PreScan Block: Path Follower){Migrate=off, FileName='Trajectory_1.mat', TunableSteeringGain=1, XShifting_wrt_COG=0}
      mask prompts: Migrate "Migrate. During migration this block will be replaced by a newer one."; FileName "Trajectory Name"; TunableSteeringGain "TunableSteeringGain [-]"; XShifting_wrt_COG "XShifting_wrt_COG [m]"
      mask help:
      | The Path Follower Model is selected in the GUI to simulate driver behavior.
      |
      | For more information, please click Help.
      mask init:
      | load(['trajectories/',eval(FileName)])
      | traject=trajectory';
      | 
      | Traj_x=traject(:,2);
      | Traj_y=traject(:,3);
      | Traj_z=traject(:,4);
      | Traj_vx=traject(:,8);
      | Traj_vy=traject(:,9);
      | Traj_vz=traject(:,10);
      mask Help: eval('openHelp(232)')
  Rate Limiter : RateLimiter  RisingSlewLimit=150  FallingSlewLimit=-150  SampleTimeMode=inherited
  SELF_Demux : Subsystem  Tag=DemuxSELF
      settings: DeleteFcn=PreScanBlockDeleteFcn;
      mask Type: PreScan Demux Block:
      mask Display:
      | port_label('output',1,'x [m]')
      | port_label('output',2,'y [m]')
      | port_label('output',3,'z [m]','texmode','on')
      | port_label('output',4,'Rotx [deg]','texmode','on')
      | port_label('output',5,'Roty [deg]','texmode','on')
      | port_label('output',6,'Rotz [deg]','texmode','on')
      | port_label('output',7,'GPS lat [deg]','texmode','on')
      | port_label('output',8,'GPS long [deg]','texmode','on')
      | port_label('output',9,'GPS alt [m]','texmode','on')
      | port_label('output',10,'Velocity [m/s]')
      | port_label('output',11,'Heading [deg]')
      | port_label('output',12,'Yaw rate [deg/s]')
  STOP Condition : Subsystem
  TSR System : ModelReference  ModelNameDialog=TSR_System  SimulationMode=Normal  ModelReferenceVersion=1.824  CopyOfModelName=TSR_System
  Terminator_{1..10} (10 alike) : Terminator
  Trajectories : Subsystem  Tag=Trajectories
      settings: DeleteFcn=PreScanBlockDeleteFcn;
      mask Type: PreScan Source Block: Trajectories
      mask Description:
      | The Trajectory block contains the trajectories defined in the PreScan Experiment Editor. The output of the trajectory block is the (vehicle) State.
      | 
      | For more information, please click Help.
      mask Help: eval('openHelp(312)')
      mask Display: image(imread('Trajectory.png'));
  Unit Delay : UnitDelay  SampleTime=-1
  Unit Delay1 : UnitDelay  SampleTime=-1
  Unit Delay2 : UnitDelay  SampleTime=-1
  VISUHeadLightLeftHBLB_Mux : Subsystem  Tag=MuxLights
      settings: DeleteFcn=PreScanBlockDeleteFcn;
      mask Type: PreScan Mux Block:
  VISUHeadLightRightHBLB_Mux : Subsystem  Tag=MuxLights
      settings: DeleteFcn=PreScanBlockDeleteFcn;
      mask Type: PreScan Mux Block:
  VISULightSource_Mux : Subsystem  Tag=MuxLightSource
      settings: DeleteFcn=PreScanBlockDeleteFcn;
      mask Type: PreScan Mux Block:
  VISUSteer_Mux : Subsystem  Tag=MuxSteer
      settings: DeleteFcn=PreScanBlockDeleteFcn;
      mask Type: PreScan Mux Block:
  VISUWheels_Mux : Subsystem  Tag=MuxWheels  mask(PreScan Mux Block:){TimeStep=1/100}
      mask prompts: TimeStep "Auto Assigned: Time Step [s]"
      settings: DeleteFcn=PreScanBlockDeleteFcn;
  pos : Constant  Tag=pos  Value=[-413.08909402600443 672.31264940005644 19.15644857361562]
  vel : Constant  Tag=pos  Value=25
  STATE_Audi_A8_1 : Outport  Tag=StateOutport
  VISULightSource_Audi_A8_1 : Outport  Tag=VisuLightsOutport  Port=2  SampleTime=1/100
  VISUWheels_Audi_A8_1 : Outport  Tag=VisuWheelsOutport  Port=3  SampleTime=1/100
  VISUSteer_Audi_A8_1 : Outport  Tag=VisuSteerOutport  Port=4  SampleTime=1/100
  VISUHeadLightRightHBLB_Audi_A8_1 : Outport  Tag=VisuHeadLightRightHBLBOutport  Port=5  SampleTime=1/100
  VISUHeadLightLeftHBLB_Audi_A8_1 : Outport  Tag=VisuHeadLightLeftHBLBOutport  Port=6  SampleTime=1/100
  tag scope: State=global
  wires:
  Compare To Constant/1 -> Data Type Conversion/1
  TSR System/1 -> Rate Limiter/1
  TSR System/2 -> [Throttle_out]
  TSR System/3 -> Terminator_10/1
  Rate Limiter/1 -> [Brake_out]
  [Rotx] -> " "/1(rotX [deg])
  [Roty] -> " "/2(rotY [deg])
  [Brake_out] -> Unit Delay/1
  Unit Delay/1 -> Compare To Constant/1
  [Steer] -> Unit Delay1/1
  Unit Delay1/1 -> Gain2/1
  [Steer] -> Unit Delay2/1
  Unit Delay2/1 -> Gain1/1
  [Params] -> Bus Selector/1
  ISA switch/1 -> TSR System/8
  [Brake_in] -> TSR System/6
  Bus Selector/1 -> TSR System/5  "<NEngine_[rpm]>"
  [Throttle_in] -> TSR System/7
  pos/1 -> PathFollower_1/1(TrajOffset_x,y,Y [m,m,deg])
  SELF_Audi_A8_1/1 -> SELF_Demux/1(SELF)
  CameraSensor_1_CM_Demux/1 -> CameraSensor_1_CM_Display/1, TSR System/2
  CameraSensor_1_CM_Demux/2 -> CameraSensor_1_CM_Display/2, TSR System/3
  CameraSensor_1_CM_Demux/3 -> CameraSensor_1_CM_Display/3, TSR System/4
  CameraSensor_1/1 -> CameraSensor_1_CM_Demux/1
  VISULightSource_Mux/1(Lights) -> VISULightSource_Audi_A8_1/1
  VISUWheels_Mux/1(Wheels) -> VISUWheels_Audi_A8_1/1
  VISUSteer_Mux/1(Steer) -> VISUSteer_Audi_A8_1/1
  VISUHeadLightRightHBLB_Mux/1(Lights) -> VISUHeadLightRightHBLB_Audi_A8_1/1
  HeadLightRightHBLB_mscd/1 -> VISUHeadLightRightHBLB_Mux/1(MSCD [Cd])
  HeadLightRightHBLB_Pos/1 -> VISUHeadLightRightHBLB_Mux/2(Position (xyz) [m])
  HeadLightRightHBLB_Ori/1 -> VISUHeadLightRightHBLB_Mux/3(Orientation (RPY) [deg])
  HeadLightRightHBLB_Col/1 -> VISUHeadLightRightHBLB_Mux/4(Color [-])
  HeadLightRightHBLB_ID/1 -> VISUHeadLightRightHBLB_Mux/5(TextureResourceID [-])
  VISUHeadLightLeftHBLB_Mux/1(Lights) -> VISUHeadLightLeftHBLB_Audi_A8_1/1
  HeadLightLeftHBLB_mscd/1 -> VISUHeadLightLeftHBLB_Mux/1(MSCD [Cd])
  HeadLightLeftHBLB_Pos/1 -> VISUHeadLightLeftHBLB_Mux/2(Position (xyz) [m])
  HeadLightLeftHBLB_Ori/1 -> VISUHeadLightLeftHBLB_Mux/3(Orientation (RPY) [deg])
  HeadLightLeftHBLB_Col/1 -> VISUHeadLightLeftHBLB_Mux/4(Color [-])
  HeadLightLeftHBLB_ID/1 -> VISUHeadLightLeftHBLB_Mux/5(TextureResourceID [-])
  Dynamics_Simple/2(Vx [m s-1]) -> [V_ms]
  PathFollower_1/2(throttle [%]) -> [Throttle_in]
  PathFollower_1/3(brake pressure [bar]) -> [Brake_in]
  PathFollower_1/4(v0 [m/s]) -> Dynamics_Simple/4(Initial_Vx_[ms-1])
  PathFollower_1/5(Auto_GearShift) -> Dynamics_Simple/6(Auto_GearShift)
  Ground_12/1 -> Dynamics_Simple/7(Manual_GearShift)
  Ground_11/1 -> VISUWheels_Mux/2(Steer Angle Rear [deg])
  Dynamics_Simple/3(Perf_Params) -> [Params]
  SELF_Demux/5(roty [deg]) -> [Roty]
  SELF_Demux/4(rotx [deg]) -> [Rotx]
  Gain1/1 -> VISUSteer_Mux/2(Steer [deg])
  Col/1 -> VISUSteer_Mux/1(Column [deg])
  " "/4(zDisp RR [m]) -> VISUWheels_Mux/7(zDisp RR [m])
  " "/3(zDisp RL [m]) -> VISUWheels_Mux/6(zDisp RL [m])
  " "/2(zDisp FR [m]) -> VISUWheels_Mux/5(zDisp FR [m])
  " "/1(zDisp FL [m]) -> VISUWheels_Mux/4(zDisp FL [m])
  [V_ms] -> VISUWheels_Mux/3(Velocity [m/s])
  Gain2/1 -> VISUWheels_Mux/1(Steer Angle Front [deg])
  Data Type Conversion/1 -> VISULightSource_Mux/9(BrakeLightLeft), VISULightSource_Mux/10(BrakeLightRight)
  [Brake_out] -> Dynamics_Simple/3(Brake)
  [Throttle_out] -> Dynamics_Simple/2(Throttle)
  PathFollower_1/1(delta_steerwheel [deg]) -> Dynamics_Simple/1(DeltaSteer_[deg]), [Steer]
  Dynamics_Simple/1(State) -> STATE_Audi_A8_1/1, [State]
  SELF_Demux/6(rotz [deg]) -> Mux/3
  SELF_Demux/1(x [m]) -> Mux/1
  SELF_Demux/2(y [m]) -> Mux/2
  Mux/1 -> PathFollower_1/3(position x,y,Y [m,m,deg])
  vel/1 -> PathFollower_1/4(Initial Velocity [m/s]), PathFollower_1/5(Desired Velocity [m/s])
  SELF_Demux/10(velocity [m/s]) -> PathFollower_1/6(velocity [m/s]), STOP Condition/1(In1), TSR System/1
  Ground_1/1 -> Dynamics_Simple/5(AutoManual_OnOff)
  Ground_2/1 -> PathFollower_1/2(ActorOffset_Left(+) / Right(-) [m])
  PathFollower_1/6(Actor/Traj_distance [m]) -> Terminator_1/1
  PathFollower_1/7(Actor/Traj_angle [deg]) -> Terminator_2/1
  SELF_Demux/3(z [m]) -> Terminator_3/1
  SELF_Demux/7(GPS lat [deg]) -> Terminator_4/1
  SELF_Demux/8(GPS long [deg]) -> Terminator_5/1
  SELF_Demux/9(GPS alt [m]) -> Terminator_6/1
  SELF_Demux/11(heading [deg]) -> Terminator_7/1
  SELF_Demux/12(yaw rate [deg/s]) -> Terminator_8/1
  Trajectories/1(State) -> Terminator_9/1
  Ground_3/1 -> VISULightSource_Mux/1(IndicatorLightsLeft)
  Ground_4/1 -> VISULightSource_Mux/2(IndicatorLightsRight)
  Ground_5/1 -> VISULightSource_Mux/3(FogLightRearLeft)
  Ground_6/1 -> VISULightSource_Mux/4(FogLightRearRight)
  Ground_7/1 -> VISULightSource_Mux/5(FogLightFrontLeft)
  Ground_8/1 -> VISULightSource_Mux/6(FogLightFrontRight)
  Ground_9/1 -> VISULightSource_Mux/7(MainLightRearLeft)
  Ground_10/1 -> VISULightSource_Mux/8(MainLightRearRight)
